simulink model "DABfull"  (R2021a)
settings: Solver=VariableStepAuto  StartTime=0.0  StopTime=10.0  RelTol=1e-3
undefined symbols (not defined in the file or in its folder): plecs
settings Model: Creator=dcostine  LastModifiedBy=dcostine

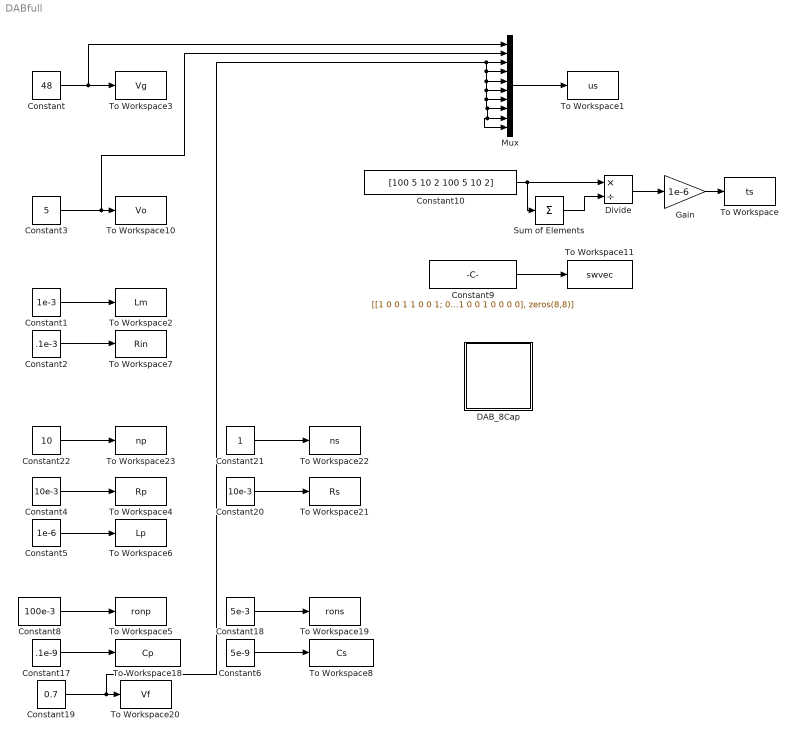
== system DABfull ==
  Constant : Constant  Value=48
  Constant1 : Constant  Value=1e-3
  Constant10 : Constant  Value=[100 5 10 2 100 5 10 2]
  Constant17 : Constant  Value=.1e-9
  Constant18 : Constant  Value=5e-3
  Constant19 : Constant  Value=0.7
  Constant2 : Constant  Value=.1e-3
  Constant20 : Constant  Value=10e-3
  Constant21 : Constant
  Constant22 : Constant  Value=10
  Constant3 : Constant  Value=5
  Constant4 : Constant  Value=10e-3
  Constant5 : Constant  Value=1e-6
  Constant6 : Constant  Value=5e-9
  Constant8 : Constant  Value=100e-3
  Constant9 : Constant  Value=[[1 0 0 1 1 0 0 1; 0 0 0 0 1 0 0 1; 0 1 1 0 1 0 0 1; 0 1 1 0 0 0 0 0; 0 1 1 0 0 1 1 0; 0 0 0 0 0 1 1 0; 1 0 0 1 0 1 1 0; 1 0 0 1 0 0 0 0], zeros(8,8)]
  DAB_8Cap : Subsystem  LoadFcn=plecs('sl', 200);  InitFcn=plecs('sl', 214);  StartFcn=plecs('sl', 208);  StopFcn=plecs('sl', 209);  mask(PlecsCircuit){PLECSData=<binary blob, 3028 chars, not shown>}
      mask prompts: PLECSData "PLECS Data (Do not delete or modify!)"
      mask init:
      | % PLACE CUSTOM INITIALIZATIONS ABOVE
      | % DO NOT REMOVE
      | plecs('sl', 215);
      | % DO NOT REMOVE
      settings: CopyFcn=plecs('sl', 203);  DeleteFcn=plecs('sl', 205);  UndoDeleteFcn=plecs('sl', 206);  PreSaveFcn=plecs('sl', 211);  PostSaveFcn=plecs('sl', 201);  NameChangeFcn=plecs('sl', 210);  DestroyFcn=plecs('sl', 207);  PreCopyFcn=plecs('sl', 216);  OpenFcn=plecs('sl', 202);  ErrorFcn=plerrorfcn
      mask Help: web(['file:///' fullfile(plecsdoc, 'creatingacircuit.html')])
      mask Display: disp('PLECS\nCircuit')
  Divide : Product  Inputs=*/
  Gain : Gain  Gain=1e-6
  Mux : Mux  Inputs=10
  Sum of Elements : Sum  Inputs=+
  To Workspace : ToWorkspace  VariableName=ts  SampleTime=-1
  To Workspace1 : ToWorkspace  VariableName=us  SampleTime=-1
  To Workspace10 : ToWorkspace  VariableName=Vo  SampleTime=-1
  To Workspace11 : ToWorkspace  VariableName=swvec  SampleTime=-1
  To Workspace18 : ToWorkspace  VariableName=Cp  SampleTime=-1
  To Workspace19 : ToWorkspace  VariableName=rons  SampleTime=-1
  To Workspace2 : ToWorkspace  VariableName=Lm  SampleTime=-1
  To Workspace20 : ToWorkspace  VariableName=Vf  SampleTime=-1
  To Workspace21 : ToWorkspace  VariableName=Rs  SampleTime=-1
  To Workspace22 : ToWorkspace  VariableName=ns  SampleTime=-1
  To Workspace23 : ToWorkspace  VariableName=np  SampleTime=-1
  To Workspace3 : ToWorkspace  VariableName=Vg  SampleTime=-1
  To Workspace4 : ToWorkspace  VariableName=Rp  SampleTime=-1
  To Workspace5 : ToWorkspace  VariableName=ronp  SampleTime=-1
  To Workspace6 : ToWorkspace  VariableName=Lp  SampleTime=-1
  To Workspace7 : ToWorkspace  VariableName=Rin  SampleTime=-1
  To Workspace8 : ToWorkspace  VariableName=Cs  SampleTime=-1
  wires:
  Constant5/1 -> To Workspace6/1
  Constant17/1 -> To Workspace18/1
  Constant/1 -> Mux/1, To Workspace3/1
  Constant3/1 -> Mux/2, To Workspace10/1
  Constant19/1 -> Mux/4, Mux/9, Mux/10, Mux/8, Mux/7, Mux/6, Mux/5, Mux/3, To Workspace20/1
  Constant8/1 -> To Workspace5/1
  Constant1/1 -> To Workspace2/1
  Constant9/1 -> To Workspace11/1
  Constant4/1 -> To Workspace4/1
  Mux/1 -> To Workspace1/1
  Constant6/1 -> To Workspace8/1
  Constant18/1 -> To Workspace19/1
  Constant20/1 -> To Workspace21/1
  Constant22/1 -> To Workspace23/1
  Constant21/1 -> To Workspace22/1
  Constant10/1 -> Divide/1, Sum of Elements/1
  Sum of Elements/1 -> Divide/2
  Divide/1 -> Gain/1
  Gain/1 -> To Workspace/1
  Constant2/1 -> To Workspace7/1

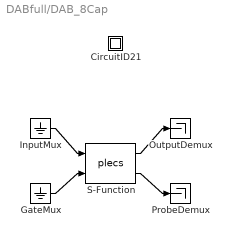
== system DABfull/DAB_8Cap ==
  " CircuitID21 " : Subsystem
  " GateMux " : Ground
  " InputMux " : Ground
  " OutputDemux " : Terminator
  " ProbeDemux " : Terminator
  " S-Function " : S-Function  FunctionName=plecs  SFunctionDeploymentMode=off  EnableBusSupport=off
  wires:
  " InputMux "/1 -> " S-Function "/1
  " GateMux "/1 -> " S-Function "/2
  " S-Function "/1 -> " OutputDemux "/1
  " S-Function "/2 -> " ProbeDemux "/1

== system DABfull/DAB_8Cap/ CircuitID21  ==
